simulink model "nonlinear_plant"  (R2019b)
settings: Solver=VariableStepAuto  StartTime=0.0  StopTime=10.0  RelTol=1e-3
undefined symbols (not defined in the file): g, I, k_T, l, M, thetaddot, thetadot, xddot
settings Model: Creator=lakshmi  LastModifiedBy=lakshmi

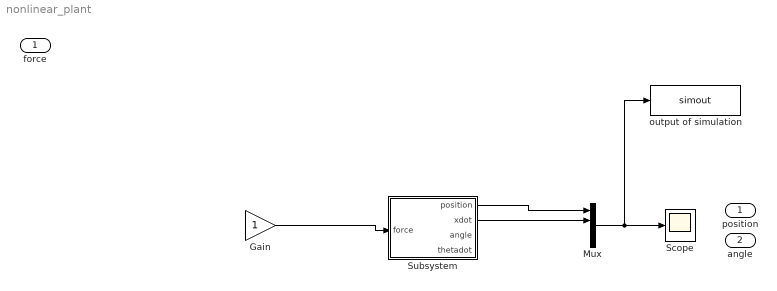
== system nonlinear_plant ==
  force : Inport
  Gain : Gain
  Mux : Mux
  Scope : Scope
  Subsystem : Subsystem
  output of simulation : ToWorkspace  VariableName=simout  SaveFormat=Timeseries  SampleTime=-1
  position : Outport
  angle : Outport  Port=2
  wires:
  Subsystem/1(position) -> Mux/1
  Subsystem/2(xdot) -> Mux/2
  Mux/1 -> output of simulation/1, Scope/1
  Gain/1 -> Subsystem/1(force)

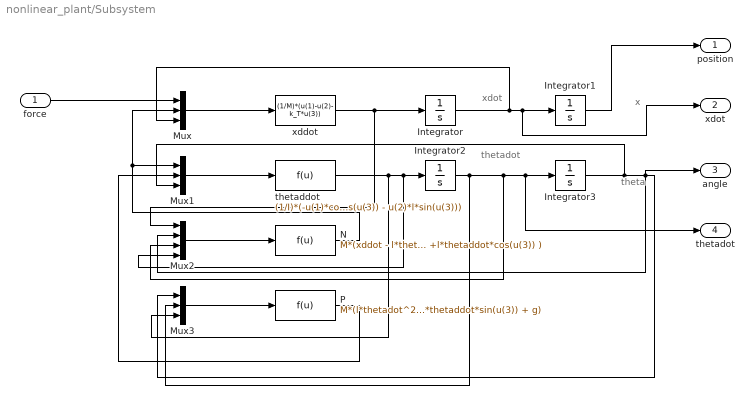
== system nonlinear_plant/Subsystem ==
  note: theta
  note: x
  note: thetadot
  note: xdot
  force : Inport
  Integrator : Integrator  ContinuousStateAttributes='xdot'
  Integrator1 : Integrator  ContinuousStateAttributes='x'
  Integrator2 : Integrator  ContinuousStateAttributes='xdot'
  Integrator3 : Integrator  InitialCondition=pi  ContinuousStateAttributes='theta'
  Mux : Mux  Inputs=3
  Mux1 : Mux  Inputs=3
  Mux2 : Mux
  Mux3 : Mux  Inputs=3
  N : Fcn  Expr=M*(xddot - l*thetadot^2*sin(u(3)) +l*thetaddot*cos(u(3)) )
  P : Fcn  Expr=M*(l*thetadot^2*cos(u(3)) + l*thetaddot*sin(u(3)) + g)
  thetaddot : Fcn  Expr=(1/I)*(-u(1)*cos(u(3)) - u(2)*l*sin(u(3)))
  "xddot " : Fcn  Expr=(1/M)*(u(1)-u(2)- k_T*u(3))
  position : Outport
  xdot : Outport  Port=2
  angle : Outport  Port=3
  thetadot : Outport  Port=4
  wires:
  P/1 -> Mux1/2
  Mux2/1 -> N/1
  thetaddot/1 -> Mux3/3, Mux2/4, Integrator2/1
  Mux/1 -> "xddot "/1
  Integrator2/1 -> Mux3/2, Mux2/3, thetadot/1, Integrator3/1
  Integrator3/1 -> Mux1/3, Mux2/2, angle/1, Mux3/1
  force/1 -> Mux/1
  Mux1/1 -> thetaddot/1
  Mux3/1 -> P/1
  Integrator1/1 -> position/1
  "xddot "/1 -> Mux2/1, Integrator/1
  Integrator/1 -> Mux/3, xdot/1, Integrator1/1
  N/1 -> Mux1/1, Mux/2
